simulink model "control_scheme"  (R2023a)
settings: Solver=VariableStepAuto  StartTime=0.0  StopTime=10.0  RelTol=1e-3
settings Model: Creator=bajdus  LastModifiedBy=bajdus

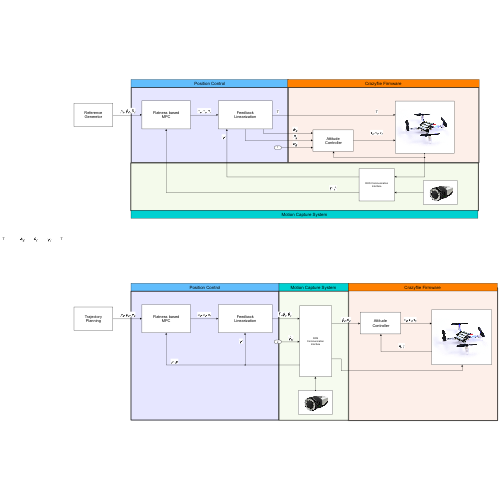
[thumbnail: Simulink's stored preview of the top-level diagram]
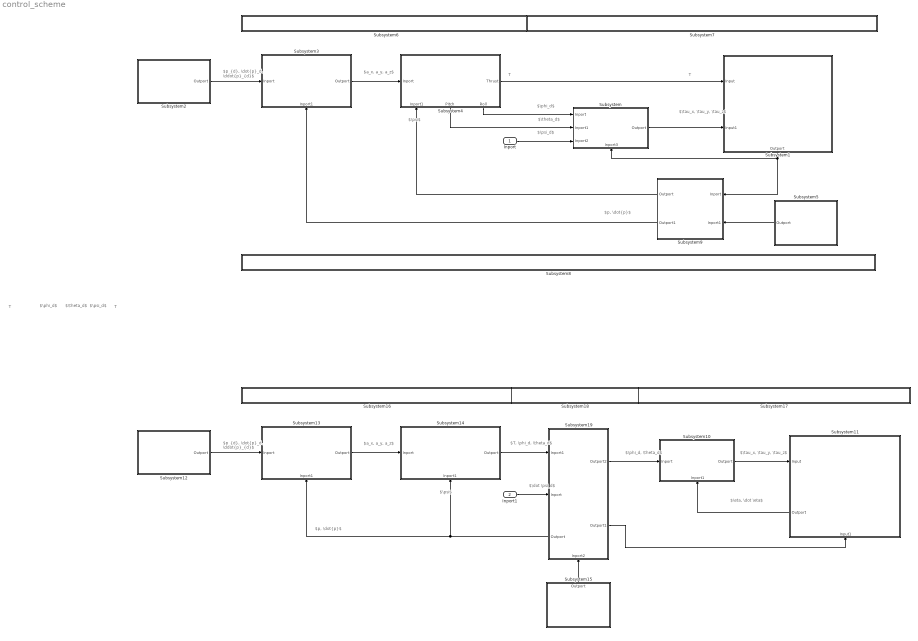
== system control_scheme ==
  note: $\dot \psi_d$
  note: $T, \phi_d, \theta_d$
  note: $\psi$
  note: $\tau_x, \tau_y, \tau_z$
  note: $\psi_d$
  note: T
  note: $\phi_d$
  note: $\theta_d$
  note: $\eta, \dot \eta$
  note: $p, \dot{p}$
  note: $p_{d}, \dot{p}_d, \ddot{p}_{d}$
  note: $a_x, a_y, a_z$
  note: T
  note: T
  note: $\tau_x, \tau_y, \tau_z$
  note: $\psi_d$
  note: T
  note: $p, \dot{p}$
  note: $\theta_d$
  note: $\phi_d$
  note: $\psi$
  note: $p_{d}, \dot{p}_d, \ddot{p}_{d}$
  note: $a_x, a_y, a_z$
  note: $\phi_d, \theta_d$
  Inport : Inport
  Inport1 : Inport  Port=2
  Subsystem : Subsystem
      settings: PortSchema="{\"entries\":[{\"content\":{\"sides\":[{\"content\":{\"connectorIds\":[\"In1\",\"In2\",\"In3\"]},\"type\":\"ConnectorPlacement.EquallySpacedRectSide\",\"uuid\":\"c4077007-7b12-41c2-8a1d-0647143a8f23\"},{\"content\":{\"connectorIds\":[\"Out1\"],\"side\":\"RIGHT\"},\"type\":\"ConnectorPlacement.EquallySpacedRectSide\",\"uuid\":\"3a1fdb27-a447-4b3a-bec9-0b15322d22a1\"},{\"content\":{\"side\":\"TOP\"},\"type\":\"ConnectorPlacement.EquallySpacedRectSide\",\"uuid\":\"adcbc497-ad35-4a74-ad13-5e823b222d1a\"},{\"content\":{\"connectorIds\":[\"In4\"],\"side\":\"BOTTOM\"},\"type\":\"ConnectorPlacement.EquallySpacedRectSide\",\"uuid\":\"f9fa7436-d207-490d-b064-e95fa0c81253\"}]},\"type\":\"ConnectorPlacement.EquallySpacedConnector\",\"uuid\":\"b00b323e-7df7-4023-ade0-db11e2c6d34f\"}],\"packageUris\":[\"http://schema.mathworks.com/mf0/Connector/R2020b\"],\"version\":\"1.0\"}"
      mask Display:
      | disp('Attitude\n');
      | disp('\n Controller');
      | % port_label('input', 1, 'u');
      | % port_label('output', 1, 'y');
      | % port_label('input', 1, 'Thrust');
      | % port_label('input', 2, 'Roll');
      | % port_label('input', 3, 'Pitch');
  Subsystem1 : Subsystem
      settings: PortSchema="{\"entries\":[{\"content\":{\"sides\":[{\"content\":{\"connectorIds\":[\"In1\",\"In2\"]},\"type\":\"ConnectorPlacement.EquallySpacedRectSide\",\"uuid\":\"4e8a3a60-2859-4132-b368-be6664223ced\"},{\"content\":{\"side\":\"RIGHT\"},\"type\":\"ConnectorPlacement.EquallySpacedRectSide\",\"uuid\":\"91531ed3-c54a-45b8-8b79-0ea378506ab7\"},{\"content\":{\"side\":\"TOP\"},\"type\":\"ConnectorPlacement.EquallySpacedRectSide\",\"uuid\":\"04ec13bb-a834-422f-bb3a-86357537ddad\"},{\"content\":{\"connectorIds\":[\"Out1\"],\"side\":\"BOTTOM\"},\"type\":\"ConnectorPlacement.EquallySpacedRectSide\",\"uuid\":\"207caced-73e4-4369-a49c-6be461eb6274\"}]},\"type\":\"ConnectorPlacement.EquallySpacedConnector\",\"uuid\":\"5d62204d-8254-4fc4-b5e1-856468f92cdd\"}],\"packageUris\":[\"http://schema.mathworks.com/mf0/Connector/R2020b\"],\"version\":\"1.0\"}"
      mask Display:
      | image('C:\Users\bajdus\Downloads\cf_21.jpg')
      | % port_label('input', 1, 'u');
      | % port_label('input', 2, 'y');
  Subsystem10 : Subsystem
      settings: PortSchema="{\"entries\":[{\"content\":{\"sides\":[{\"content\":{\"connectorIds\":[\"In1\"]},\"type\":\"ConnectorPlacement.EquallySpacedRectSide\",\"uuid\":\"4e8a3a60-2859-4132-b368-be6664223ced\"},{\"content\":{\"connectorIds\":[\"Out1\"],\"side\":\"RIGHT\"},\"type\":\"ConnectorPlacement.EquallySpacedRectSide\",\"uuid\":\"91531ed3-c54a-45b8-8b79-0ea378506ab7\"},{\"content\":{\"side\":\"TOP\"},\"type\":\"ConnectorPlacement.EquallySpacedRectSide\",\"uuid\":\"04ec13bb-a834-422f-bb3a-86357537ddad\"},{\"content\":{\"connectorIds\":[\"In2\"],\"side\":\"BOTTOM\"},\"type\":\"ConnectorPlacement.EquallySpacedRectSide\",\"uuid\":\"272fcaa4-9016-4ded-b571-18b09d4b29f1\"}]},\"type\":\"ConnectorPlacement.EquallySpacedConnector\",\"uuid\":\"5d62204d-8254-4fc4-b5e1-856468f92cdd\"}],\"packageUris\":[\"http://schema.mathworks.com/mf0/Connector/R2020b\"],\"version\":\"1.0\"}"
      mask Display:
      | disp('Attitude\n');
      | disp('\n Controller');
      | % port_label('input', 1, 'u');
      | % port_label('output', 1, 'y');
      | % port_label('input', 1, 'Thrust');
      | % port_label('input', 2, 'Roll');
      | % port_label('input', 3, 'Pitch');
  Subsystem11 : Subsystem
      settings: PortSchema="{\"entries\":[{\"content\":{\"sides\":[{\"content\":{\"connectorIds\":[\"In1\",\"Out1\"]},\"type\":\"ConnectorPlacement.EquallySpacedRectSide\",\"uuid\":\"4e8a3a60-2859-4132-b368-be6664223ced\"},{\"content\":{\"side\":\"RIGHT\"},\"type\":\"ConnectorPlacement.EquallySpacedRectSide\",\"uuid\":\"91531ed3-c54a-45b8-8b79-0ea378506ab7\"},{\"content\":{\"side\":\"TOP\"},\"type\":\"ConnectorPlacement.EquallySpacedRectSide\",\"uuid\":\"04ec13bb-a834-422f-bb3a-86357537ddad\"},{\"content\":{\"connectorIds\":[\"In2\"],\"side\":\"BOTTOM\"},\"type\":\"ConnectorPlacement.EquallySpacedRectSide\",\"uuid\":\"207caced-73e4-4369-a49c-6be461eb6274\"}]},\"type\":\"ConnectorPlacement.EquallySpacedConnector\",\"uuid\":\"5d62204d-8254-4fc4-b5e1-856468f92cdd\"}],\"packageUris\":[\"http://schema.mathworks.com/mf0/Connector/R2020b\"],\"version\":\"1.0\"}"
      mask Display:
      | image('C:\Users\bajdus\Downloads\cf_21.jpg')
      | % port_label('input', 1, 'u');
      | % port_label('input', 2, 'y');
  Subsystem12 : Subsystem
      mask Display:
      | disp('Trajectory\n');
      | disp('\nPlanning');
      | % port_label('output', 1, 'y');
  Subsystem13 : Subsystem
      settings: PortSchema="{\"entries\":[{\"content\":{\"sides\":[{\"content\":{\"connectorIds\":[\"In1\"]},\"type\":\"ConnectorPlacement.EquallySpacedRectSide\",\"uuid\":\"4e8a3a60-2859-4132-b368-be6664223ced\"},{\"content\":{\"connectorIds\":[\"Out1\"],\"side\":\"RIGHT\"},\"type\":\"ConnectorPlacement.EquallySpacedRectSide\",\"uuid\":\"91531ed3-c54a-45b8-8b79-0ea378506ab7\"},{\"content\":{\"side\":\"TOP\"},\"type\":\"ConnectorPlacement.EquallySpacedRectSide\",\"uuid\":\"04ec13bb-a834-422f-bb3a-86357537ddad\"},{\"content\":{\"connectorIds\":[\"In2\"],\"side\":\"BOTTOM\"},\"type\":\"ConnectorPlacement.EquallySpacedRectSide\",\"uuid\":\"d91d8de1-f07e-4685-9794-dc78f6f14931\"}]},\"type\":\"ConnectorPlacement.EquallySpacedConnector\",\"uuid\":\"5d62204d-8254-4fc4-b5e1-856468f92cdd\"}],\"packageUris\":[\"http://schema.mathworks.com/mf0/Connector/R2020b\"],\"version\":\"1.0\"}"
      mask Display:
      | disp('Flatness based\n');
      | disp('\nMPC');
      | % port_label('input', 1, 'u');
      | % port_label('output', 1, 'y');
  Subsystem14 : Subsystem
      settings: PortSchema="{\"entries\":[{\"content\":{\"sides\":[{\"content\":{\"connectorIds\":[\"In1\"]},\"type\":\"ConnectorPlacement.EquallySpacedRectSide\",\"uuid\":\"c8c5d0ec-bac6-4776-ab4b-3252e9617757\"},{\"content\":{\"connectorIds\":[\"Out1\"],\"side\":\"RIGHT\"},\"type\":\"ConnectorPlacement.EquallySpacedRectSide\",\"uuid\":\"083abae2-ef28-470e-845d-5e065b7c2f13\"},{\"content\":{\"side\":\"TOP\"},\"type\":\"ConnectorPlacement.EquallySpacedRectSide\",\"uuid\":\"1d4c5a5f-3dac-4657-9352-c2a171996430\"},{\"content\":{\"connectorIds\":[\"In2\"],\"side\":\"BOTTOM\"},\"type\":\"ConnectorPlacement.EquallySpacedRectSide\",\"uuid\":\"55b6361b-daf7-4dc1-9809-c37205559468\"}]},\"type\":\"ConnectorPlacement.EquallySpacedConnector\",\"uuid\":\"51f478ca-b7f9-4d90-9059-a531f3bd74ef\"}],\"packageUris\":[\"http://schema.mathworks.com/mf0/Connector/R2020b\"],\"version\":\"1.0\"}"
      mask Display:
      | disp('Feedback\n');
      | disp('\nLinearization');
      | % port_label('input', 1, 'u');
      | % port_label('output', 1, 'y');
      | 
      | % port_label('output', 1, 'Thrust');
      | % port_label('output', 2, 'Roll');
      | % port_label('output', 3, 'Pitch');
  Subsystem15 : Subsystem
      settings: PortSchema="{\"entries\":[{\"content\":{\"sides\":[{\"content\":{},\"type\":\"ConnectorPlacement.EquallySpacedRectSide\",\"uuid\":\"349d1282-79b4-46c7-8fc5-7d6e6dda5074\"},{\"content\":{\"side\":\"RIGHT\"},\"type\":\"ConnectorPlacement.EquallySpacedRectSide\",\"uuid\":\"2ee40947-3749-41aa-98b7-cce664f53032\"},{\"content\":{\"connectorIds\":[\"Out1\"],\"side\":\"TOP\"},\"type\":\"ConnectorPlacement.EquallySpacedRectSide\",\"uuid\":\"0fcae5b9-bd41-44ff-813f-2af407d400d3\"}]},\"type\":\"ConnectorPlacement.EquallySpacedConnector\",\"uuid\":\"b417121a-f176-4ed3-a85c-8909c3dffad0\"}],\"packageUris\":[\"http://schema.mathworks.com/mf0/Connector/R2020b\"],\"version\":\"1.0\"}"
      mask Display:
      | image('C:\Users\bajdus\Downloads\miqus_cam.jpeg')
      | % port_label('input', 1, 'u');
      | % port_label('input', 2, 'y');
  Subsystem16 : Subsystem
      mask Display: disp("Position Control");
  Subsystem17 : Subsystem
      mask Display: disp("Crazyflie Firmware");
  Subsystem18 : Subsystem
      mask Display: disp("Motion Capture System");
  Subsystem19 : Subsystem
      settings: PortSchema="{\"entries\":[{\"content\":{\"sides\":[{\"content\":{\"connectorIds\":[\"Out2\",\"Out3\"]},\"type\":\"ConnectorPlacement.EquallySpacedRectSide\",\"uuid\":\"451318d0-1f43-4408-9f5f-a46949c009ff\"},{\"content\":{\"connectorIds\":[\"Out1\",\"In2\",\"In3\"],\"side\":\"RIGHT\"},\"type\":\"ConnectorPlacement.EquallySpacedRectSide\",\"uuid\":\"3a3251aa-9aee-4f6c-93a9-eae1e8871d77\"},{\"content\":{\"connectorIds\":[\"In1\"],\"side\":\"TOP\"},\"type\":\"ConnectorPlacement.EquallySpacedRectSide\",\"uuid\":\"e6eb2623-8557-4c01-8a0c-835f970dce30\"}]},\"type\":\"ConnectorPlacement.EquallySpacedConnector\",\"uuid\":\"025b3b78-9819-4a0e-919f-681470b94be9\"}],\"packageUris\":[\"http://schema.mathworks.com/mf0/Connector/R2020b\"],\"version\":\"1.0\"}"
      mask Display:
      | % disp('ROS Communication\n');
      | % disp('\nInterface')
      | 
      | disp('ROS\nCommunication\nInterface');
  Subsystem2 : Subsystem
      mask Display:
      | disp('Reference\n');
      | disp('\nGeneretor');
      | % port_label('output', 1, 'y');
  Subsystem3 : Subsystem
      settings: PortSchema="{\"entries\":[{\"content\":{\"sides\":[{\"content\":{\"connectorIds\":[\"In1\"]},\"type\":\"ConnectorPlacement.EquallySpacedRectSide\",\"uuid\":\"4e8a3a60-2859-4132-b368-be6664223ced\"},{\"content\":{\"connectorIds\":[\"Out1\"],\"side\":\"RIGHT\"},\"type\":\"ConnectorPlacement.EquallySpacedRectSide\",\"uuid\":\"91531ed3-c54a-45b8-8b79-0ea378506ab7\"},{\"content\":{\"side\":\"TOP\"},\"type\":\"ConnectorPlacement.EquallySpacedRectSide\",\"uuid\":\"04ec13bb-a834-422f-bb3a-86357537ddad\"},{\"content\":{\"connectorIds\":[\"In2\"],\"side\":\"BOTTOM\"},\"type\":\"ConnectorPlacement.EquallySpacedRectSide\",\"uuid\":\"d91d8de1-f07e-4685-9794-dc78f6f14931\"}]},\"type\":\"ConnectorPlacement.EquallySpacedConnector\",\"uuid\":\"5d62204d-8254-4fc4-b5e1-856468f92cdd\"}],\"packageUris\":[\"http://schema.mathworks.com/mf0/Connector/R2020b\"],\"version\":\"1.0\"}"
      mask Display:
      | disp('Flatness based\n');
      | disp('\nMPC');
      | % port_label('input', 1, 'u');
      | % port_label('output', 1, 'y');
  Subsystem4 : Subsystem
      settings: PortSchema="{\"entries\":[{\"content\":{\"sides\":[{\"content\":{\"connectorIds\":[\"In1\"]},\"type\":\"ConnectorPlacement.EquallySpacedRectSide\",\"uuid\":\"c8c5d0ec-bac6-4776-ab4b-3252e9617757\"},{\"content\":{\"connectorIds\":[\"Out1\"],\"side\":\"RIGHT\"},\"type\":\"ConnectorPlacement.EquallySpacedRectSide\",\"uuid\":\"083abae2-ef28-470e-845d-5e065b7c2f13\"},{\"content\":{\"side\":\"TOP\"},\"type\":\"ConnectorPlacement.EquallySpacedRectSide\",\"uuid\":\"1d4c5a5f-3dac-4657-9352-c2a171996430\"},{\"content\":{\"connectorIds\":[\"In2\",\"Out2\",\"Out3\"],\"side\":\"BOTTOM\"},\"type\":\"ConnectorPlacement.EquallySpacedRectSide\",\"uuid\":\"55b6361b-daf7-4dc1-9809-c37205559468\"}]},\"type\":\"ConnectorPlacement.EquallySpacedConnector\",\"uuid\":\"51f478ca-b7f9-4d90-9059-a531f3bd74ef\"}],\"packageUris\":[\"http://schema.mathworks.com/mf0/Connector/R2020b\"],\"version\":\"1.0\"}"
      mask Display:
      | disp('Feedback\n');
      | disp('\nLinearization');
      | % port_label('input', 1, 'u');
      | % port_label('output', 1, 'y');
      | 
      | % port_label('output', 1, 'Thrust');
      | % port_label('output', 2, 'Roll');
      | % port_label('output', 3, 'Pitch');
  Subsystem5 : Subsystem
      mask Display:
      | image('C:\Users\bajdus\Downloads\miqus_cam.jpeg')
      | % port_label('input', 1, 'u');
      | % port_label('input', 2, 'y');
  Subsystem6 : Subsystem
      mask Display: disp("Position Control");
  Subsystem7 : Subsystem
      mask Display: disp("Crazyflie Firmware");
  Subsystem8 : Subsystem
      mask Display: disp("Motion Capture System");
  Subsystem9 : Subsystem
      settings: PortSchema="{\"entries\":[{\"content\":{\"sides\":[{\"content\":{\"connectorIds\":[\"Out1\",\"Out2\"]},\"type\":\"ConnectorPlacement.EquallySpacedRectSide\",\"uuid\":\"451318d0-1f43-4408-9f5f-a46949c009ff\"},{\"content\":{\"connectorIds\":[\"In1\",\"In2\"],\"side\":\"RIGHT\"},\"type\":\"ConnectorPlacement.EquallySpacedRectSide\",\"uuid\":\"3a3251aa-9aee-4f6c-93a9-eae1e8871d77\"},{\"content\":{\"side\":\"TOP\"},\"type\":\"ConnectorPlacement.EquallySpacedRectSide\",\"uuid\":\"e6eb2623-8557-4c01-8a0c-835f970dce30\"}]},\"type\":\"ConnectorPlacement.EquallySpacedConnector\",\"uuid\":\"025b3b78-9819-4a0e-919f-681470b94be9\"}],\"packageUris\":[\"http://schema.mathworks.com/mf0/Connector/R2020b\"],\"version\":\"1.0\"}"
      mask Display:
      | disp('ROS Communication\n');
      | disp('\nInterface')
  wires:
  Subsystem2/1(Outport) -> Subsystem3/1(Inport)
  Subsystem/1(Outport) -> Subsystem1/2(Input1)
  Subsystem3/1(Outport) -> Subsystem4/1(Inport)
  Subsystem4/1(Thrust) -> Subsystem1/1(Input)
  Subsystem4/3(Roll) -> Subsystem/1(Inport)
  Subsystem4/2(Pitch) -> Subsystem/2(Inport1)
  Inport/1 -> Subsystem/3(Inport2)
  Subsystem5/1(Outport) -> Subsystem9/2(Inport1)
  Subsystem9/2(Outport1) -> Subsystem3/2(Inport1)
  Subsystem1/1(Outport) -> Subsystem9/1(Inport), Subsystem/4(Inport3)
  Subsystem9/1(Outport) -> Subsystem4/2(Inport1)
  Subsystem12/1(Outport) -> Subsystem13/1(Inport)
  Subsystem13/1(Outport) -> Subsystem14/1(Inport)
  Subsystem14/1(Outport) -> Subsystem19/3(Inport1)
  Inport1/1 -> Subsystem19/2(Inport)
  Subsystem15/1(Outport) -> Subsystem19/1(Inport2)
  Subsystem19/3(Outport2) -> Subsystem10/1(Inport)
  Subsystem10/1(Outport) -> Subsystem11/1(Input)
  Subsystem19/2(Outport1) -> Subsystem11/2(Input1)
  Subsystem11/1(Outport) -> Subsystem10/2(Inport1)
  Subsystem19/1(Outport) -> Subsystem13/2(Inport1), Subsystem14/2(Inport1)

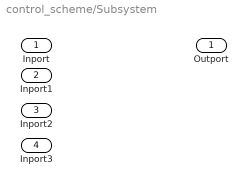
== system control_scheme/Subsystem ==
  Inport : Inport
  Inport1 : Inport  Port=2
  Inport2 : Inport  Port=3
  Inport3 : Inport  Port=4
  Outport : Outport

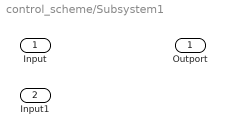
== system control_scheme/Subsystem1 ==
  Input : Inport
  Input1 : Inport  Port=2
  Outport : Outport

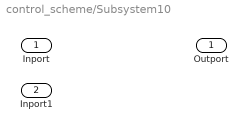
== system control_scheme/Subsystem10 ==
  Inport : Inport
  Inport1 : Inport  Port=2
  Outport : Outport

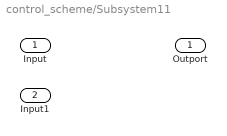
== system control_scheme/Subsystem11 ==
  Input : Inport
  Input1 : Inport  Port=2
  Outport : Outport

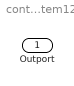
== system control_scheme/Subsystem12 ==
  Outport : Outport

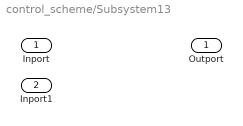
== system control_scheme/Subsystem13 ==
  Inport : Inport
  Inport1 : Inport  Port=2
  Outport : Outport

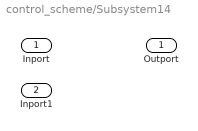
== system control_scheme/Subsystem14 ==
  Inport : Inport
  Inport1 : Inport  Port=2
  Outport : Outport

== system control_scheme/Subsystem15 ==
  Outport : Outport

== system control_scheme/Subsystem16 ==

== system control_scheme/Subsystem17 ==

== system control_scheme/Subsystem18 ==

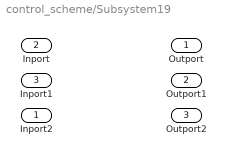
== system control_scheme/Subsystem19 ==
  Inport2 : Inport
  Inport : Inport  Port=2
  Inport1 : Inport  Port=3
  Outport : Outport
  Outport1 : Outport  Port=2
  Outport2 : Outport  Port=3

== system control_scheme/Subsystem2 ==
  Outport : Outport

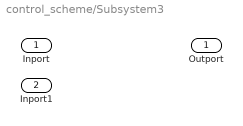
== system control_scheme/Subsystem3 ==
  Inport : Inport
  Inport1 : Inport  Port=2
  Outport : Outport

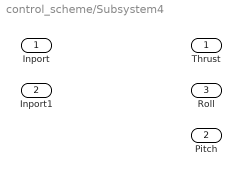
== system control_scheme/Subsystem4 ==
  Inport : Inport
  Inport1 : Inport  Port=2
  Thrust : Outport
  Pitch : Outport  Port=2
  Roll : Outport  Port=3

== system control_scheme/Subsystem5 ==
  Outport : Outport

== system control_scheme/Subsystem6 ==

== system control_scheme/Subsystem7 ==

== system control_scheme/Subsystem8 ==

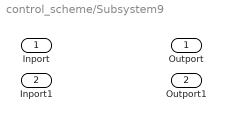
== system control_scheme/Subsystem9 ==
  Inport : Inport
  Inport1 : Inport  Port=2
  Outport : Outport
  Outport1 : Outport  Port=2
